simulink model "Lab1_419_sim7"  (R2023b)
settings: Solver=VariableStepAuto  StartTime=0.0  StopTime=270  RelTol=1e-9
undefined symbols (not defined in the file): desired
settings Model: Creator=julia  LastModifiedBy=julia

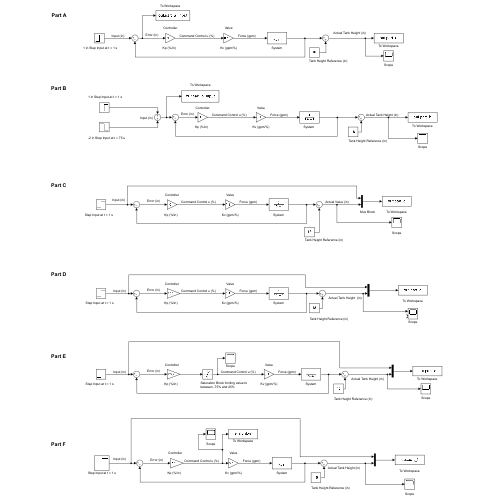
[thumbnail: Simulink's stored preview of the top-level diagram]
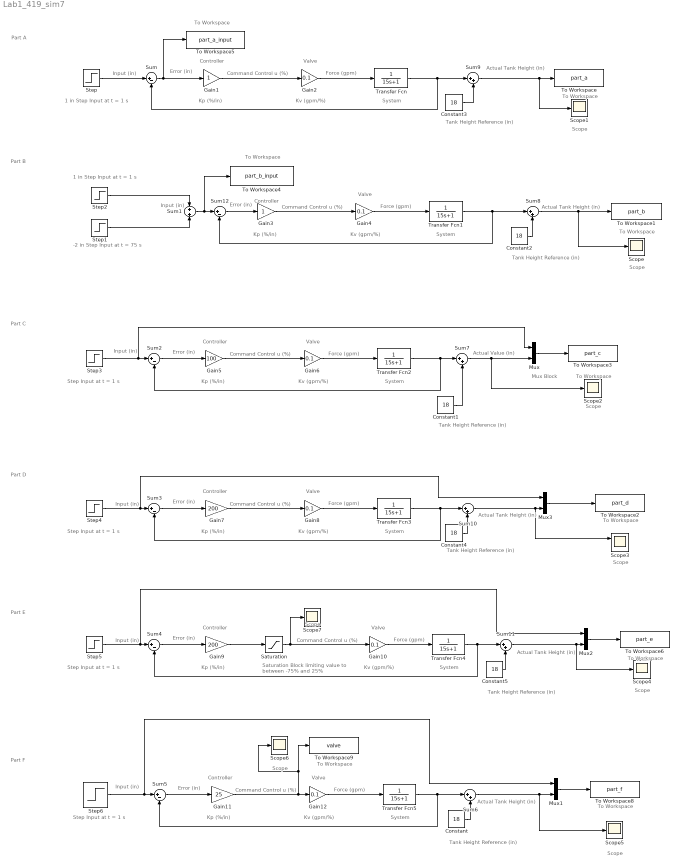
== system Lab1_419_sim7 ==
  note: Tank Height Reference (in)
  note: System
  note: Saturation Block limiting value to between -75% and 25%
  note: Scope
  note: To Workspace
  note: Actual Tank Height (in)
  note: Force (gpm)
  note: Controller
  note: Command Control u (%)
  note: Error (in)
  note: Kv (gpm/%)
  note: Valve
  note: Input (in)
  note: Kp (%/in)
  note: 1 in Step Input at t = 1 s
  note: Part A
  note: Part B
  note: Input (in)
  note: Force (gpm)
  note: Kv (gpm/%)
  note: Error (in)
  note: Actual Tank Height (in)
  note: Kp (%/in)
  note: Controller
  note: Command Control u (%)
  note: Valve
  note: 1 in Step Input at t = 1 s
  note: -2 in Step Input at t = 75 s
  note: To Workspace
  note: Scope
  note: Input (in)
  note: To Workspace
  note: Force (gpm)
  note: Error (in)
  note: Kv (gpm/%)
  note: Valve
  note: Mux Block
  note: Step Input at t = 1 s
  note: Actual Value (in)
  note: Kp (%/in)
  note: Controller
  note: Command Control u (%)
  note: Scope
  note: Part C
  note: Input (in)
  note: Valve
  note: Kv (gpm/%)
  note: Error (in)
  note: To Workspace
  note: Force (gpm)
  note: Controller
  note: Part D
  note: Command Control u (%)
  note: Kp (%/in)
  note: Scope
  note: Actual Tank Height (in)
  note: Step Input at t = 1 s
  note: Kp (%/in)
  note: Scope
  note: Command Control u (%)
  note: Step Input at t = 1 s
  note: Part E
  note: Controller
  note: Force (gpm)
  note: Input (in)
  note: Kv (gpm/%)
  note: Valve
  note: Error (in)
  note: To Workspace
  note: Kp (%/in)
  note: Scope
  note: Actual Tank Height (in)
  note: Command Control u (%)
  note: Step Input at t = 1 s
  note: To Workspace
  note: Part F
  note: Controller
  note: Force (gpm)
  note: Input (in)
  note: Kv (gpm/%)
  note: Valve
  note: Error (in)
  note: To Workspace
  note: Scope
  note: Actual Tank Height (in)
  note: Scope
  note: To Workspace
  note: To Workspace
  note: System
  note: System
  note: System
  note: System
  note: System
  note: Tank Height Reference (in)
  note: Tank Height Reference (in)
  note: Tank Height Reference (in)
  note: Tank Height Reference (in)
  note: Tank Height Reference (in)
  Constant{,1..5} (6 alike) : Constant  Value=18
  Gain1 : Gain
  Gain{2,4,6,8,10,12} (6 alike) : Gain  Gain=0.1
  Gain11 : Gain  Gain=25
  Gain3 : Gain
  Gain5 : Gain  Gain=100
  Gain7 : Gain  Gain=200
  Gain9 : Gain  Gain=200
  Mux{,1..3} (4 alike) : Mux  Inputs=2
  Saturation : Saturate  UpperLimit=25  LowerLimit=-75
  Scope{,1..2,4..7} (7 alike) : Scope
  Scope3 : Scope  NumInputPorts=2
  Step : Step  SampleTime=1
  Step1 : Step  Time=75  Before=1  After=-1  SampleTime=1
  Step2 : Step  SampleTime=1
  Step{3..6} (4 alike) : Step  After=desired-18  SampleTime=1
  Sum{,2..5,12} (6 alike) : Sum  Inputs=|+-
  Sum1 : Sum
  Sum{6..11} (6 alike) : Sum  Inputs=|++
  To Workspace : ToWorkspace  VariableName=part_a  SampleTime=-1
  To Workspace1 : ToWorkspace  VariableName=part_b  SampleTime=-1
  To Workspace2 : ToWorkspace  VariableName=part_d  SampleTime=-1
  To Workspace3 : ToWorkspace  VariableName=part_c  SampleTime=-1
  To Workspace4 : ToWorkspace  VariableName=part_b_input  SampleTime=-1
  To Workspace5 : ToWorkspace  VariableName=part_a_input  SampleTime=-1
  To Workspace6 : ToWorkspace  VariableName=part_e  SampleTime=-1
  To Workspace8 : ToWorkspace  VariableName=part_f  SampleTime=-1
  To Workspace9 : ToWorkspace  VariableName=valve  SampleTime=-1
  Transfer Fcn{,1..5} (6 alike) : TransferFcn  Denominator=[15 1]
  wires:
  Step/1 -> Sum/1
  Sum/1 -> To Workspace5/1, Gain1/1
  Gain1/1 -> Gain2/1
  Gain2/1 -> Transfer Fcn/1
  Sum1/1 -> To Workspace4/1, Sum12/1
  Gain3/1 -> Gain4/1
  Gain4/1 -> Transfer Fcn1/1
  Step1/1 -> Sum1/2
  Step2/1 -> Sum1/1
  Gain5/1 -> Gain6/1
  Sum2/1 -> Gain5/1
  Step3/1 -> Mux/1, Sum2/1
  Gain6/1 -> Transfer Fcn2/1
  Gain8/1 -> Transfer Fcn3/1
  Step4/1 -> Mux3/1, Sum3/1
  Sum3/1 -> Gain7/1
  Gain7/1 -> Gain8/1
  Gain10/1 -> Transfer Fcn4/1
  Gain9/1 -> Saturation/1
  Sum4/1 -> Gain9/1
  Saturation/1 -> Scope7/1, Gain10/1
  Transfer Fcn5/1 -> Sum6/1, Sum5/2
  Gain12/1 -> Transfer Fcn5/1
  Gain11/1 -> Scope6/1, To Workspace9/1, Gain12/1
  Sum5/1 -> Gain11/1
  Step6/1 -> Mux1/1, Sum5/1
  Constant/1 -> Sum6/2
  Mux/1 -> To Workspace3/1
  Transfer Fcn2/1 -> Sum7/1, Sum2/2
  Sum7/1 -> Scope2/1, Mux/2
  Constant1/1 -> Sum7/2
  Transfer Fcn1/1 -> Sum12/2, Sum8/1
  Sum8/1 -> Scope/1, To Workspace1/1
  Constant2/1 -> Sum8/2
  Transfer Fcn/1 -> Sum9/1, Sum/2
  Sum9/1 -> Scope1/1, To Workspace/1
  Constant3/1 -> Sum9/2
  Transfer Fcn3/1 -> Sum10/1, Sum3/2
  Constant4/1 -> Sum10/2
  Sum6/1 -> Scope5/1, Mux1/2
  Mux1/1 -> To Workspace8/1
  Constant5/1 -> Sum11/2
  Transfer Fcn4/1 -> Sum11/1, Sum4/2
  Mux2/1 -> To Workspace6/1
  Sum11/1 -> Scope4/1, Mux2/2
  Step5/1 -> Mux2/1, Sum4/1
  Sum10/1 -> Scope3/1, Mux3/2
  Mux3/1 -> To Workspace2/1
  Sum12/1 -> Gain3/1
